simulink model "gm_sfir_fixed_vnl"  (R2021b)
settings: Solver=FixedStepDiscrete  StartTime=0.0  StopTime=2000  RelTol=1e-3
libraries: simulink x2
Description:
  | Symmetric FIR Filter
  | This example shows how to use HDL Coder(TM) to check, generate,
  | and verify HDL for a fixed-point symmetric FIR filter.
settings Model: Creator=The MathWorks, Inc.  LastModifiedBy=Marco Milanesi
settings SolverCC: AlgebraicLoopSolver=TrustRegion
settings DataIOCC: LimitDataPoints=on  SaveFormat=Array  SaveOutput=off  SignalLogging=off  SaveTime=off  ReturnWorkspaceOutputs=off  SignalLoggingName=logsOut
settings OptimizationCC: BlockReduction=off  BooleanDataType=off  ConditionallyExecuteInputs=off  DefaultParameterBehavior=Inlined  InheritOutputTypeSmallerThanSingle=on  InlineInvariantSignals=on  ExpressionDepthLimit=2147483647  InitFltsAndDblsToZero=on  LifeSpan=inf  BufferReusableBoundary=off
settings DebuggingCC: AlgebraicLoopMsg=error  SaveWithParameterizedLinksMsg=none  UnderspecifiedInitializationDetection=Classic  MergeDetectMultiDrivingBlocksExec=none  CheckExecutionContextPreStartOutputMsg=on  SignalResolutionControl=TryResolveAllWithWarning  InheritedTsInSrcMsg=none  MultiTaskDSMMsg=warning  MultiTaskCondExecSysMsg=none  SingleTaskRateTransMsg=error  IntegerOverflowMsg=none  ParameterPrecisionLossMsg=none  FcnCallInpInsideContextMsg=warning  BusObjectLabelMismatch=none  StateNameClashWarn=warning  SFUnexpectedBacktrackingDiag=warning  SFNoUnconditionalDefaultTransitionDiag=warning  SFExecutionAtInitializationDiag=none  SFMachineParentedDataDiag=warning  IntegerSaturationMsg=none  ArithmeticOperatorsInVariantConditions=warning
settings HardwareCC: ProdBitPerPointer=32  ProdBitPerSizeT=32  ProdBitPerPtrDiffT=32  ProdLargestAtomicFloat=None  ProdIntDivRoundTo=Undefined  ProdEndianess=Unspecified  ProdWordSize=32  ProdHWDeviceType=ASIC/FPGA  TargetUnknown=on  ProdEqTarget=off
settings ModelReferenceCC: PropagateSignalLabelsOutOfModel=off
settings SFSimCC: SimUseLocalCustomCode=off  CustomCodeUndefinedFunction=UseInterfaceOnly
settings RTWCC: RTWUseLocalCustomCode=off
settings CodeAppCC: StateflowObjectComments=on
settings GRTTargetCC: TargetFcnLib=ansi_tfl_tmw.mat  TargetLangStandard=C89/C90 (ANSI)  CombineOutputUpdateFcns=off  GRTInterface=on
settings ConfigComp: CovMetricSettings=dw  CovSaveCumulativeToWorkspaceVar=on  CovSaveSingleToWorkspaceVar=on  CovExternalEMLEnable=off

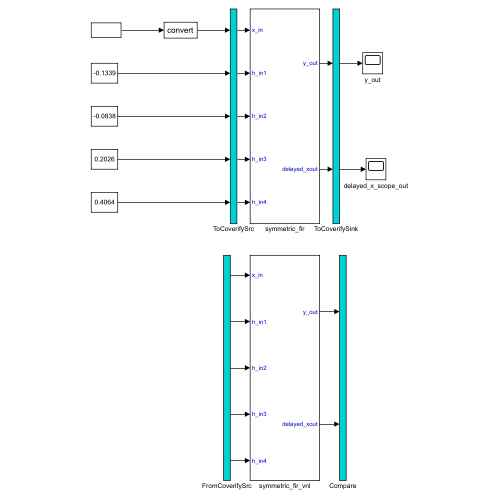
[thumbnail: Simulink's stored preview of the top-level diagram]
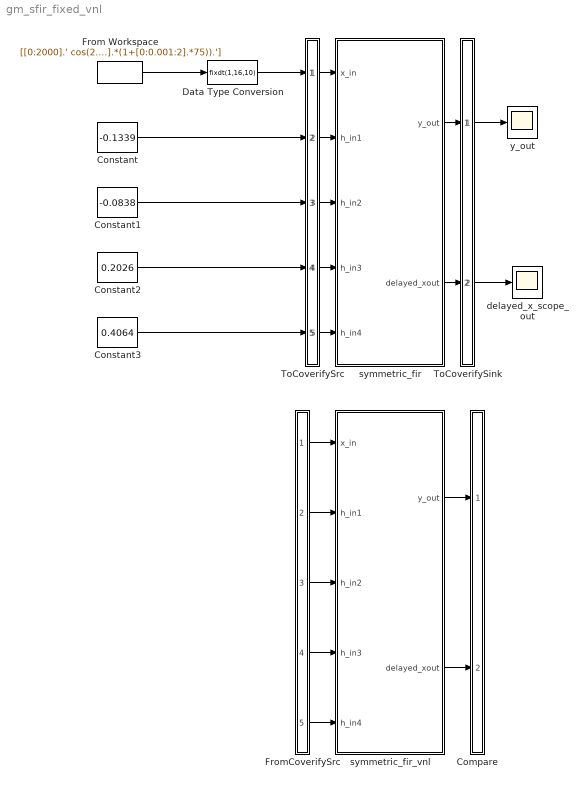
== system gm_sfir_fixed_vnl ==
  Compare : Subsystem
      mask Display: disp('')
  Constant : Constant  Value=-0.1339  OutDataTypeStr=fixdt(1,16,10)  SampleTime=1
  Constant1 : Constant  Value=-0.0838  OutDataTypeStr=fixdt(1,16,10)  SampleTime=1
  Constant2 : Constant  Value=0.2026  OutDataTypeStr=fixdt(1,16,10)  SampleTime=1
  Constant3 : Constant  Value=0.4064  OutDataTypeStr=fixdt(1,16,10)  SampleTime=1
  Data Type Conversion : DataTypeConversion  OutDataTypeStr=fixdt(1,16,10)
  From Workspace : FromWorkspace  VariableName=[[0:2000].' cos(2.*pi.*[0:0.001:2].*(1+[0:0.001:2].*75)).']  SampleTime=1  OutputAfterFinalValue=Setting to zero
  FromCoverifySrc : Subsystem
      mask Display: disp('')
  ToCoverifySink : Subsystem
      mask Display: disp('')
  ToCoverifySrc : Subsystem
      mask Display: disp('')
  delayed_x_scope_out : Scope
  symmetric_fir : Subsystem
  symmetric_fir_vnl : Subsystem
  y_out : Scope
  wires:
  From Workspace/1 -> Data Type Conversion/1
  ToCoverifySrc/1(out1) -> symmetric_fir/1(x_in)
  ToCoverifySrc/2(out2) -> symmetric_fir/2(h_in1)
  ToCoverifySrc/3(out3) -> symmetric_fir/3(h_in2)
  ToCoverifySrc/4(out4) -> symmetric_fir/4(h_in3)
  ToCoverifySrc/5(out5) -> symmetric_fir/5(h_in4)
  symmetric_fir/1(y_out) -> ToCoverifySink/1(in1)
  symmetric_fir/2(delayed_xout) -> ToCoverifySink/2(in2)
  Data Type Conversion/1 -> ToCoverifySrc/1(in1)
  Constant/1 -> ToCoverifySrc/2(in2)
  Constant1/1 -> ToCoverifySrc/3(in3)
  Constant2/1 -> ToCoverifySrc/4(in4)
  Constant3/1 -> ToCoverifySrc/5(in5)
  ToCoverifySink/1(out1) -> y_out/1
  ToCoverifySink/2(out2) -> delayed_x_scope_out/1
  FromCoverifySrc/1(out1) -> symmetric_fir_vnl/1(x_in)
  FromCoverifySrc/2(out2) -> symmetric_fir_vnl/2(h_in1)
  FromCoverifySrc/3(out3) -> symmetric_fir_vnl/3(h_in2)
  FromCoverifySrc/4(out4) -> symmetric_fir_vnl/4(h_in3)
  FromCoverifySrc/5(out5) -> symmetric_fir_vnl/5(h_in4)
  symmetric_fir_vnl/1(y_out) -> Compare/1(in1)
  symmetric_fir_vnl/2(delayed_xout) -> Compare/2(in2)

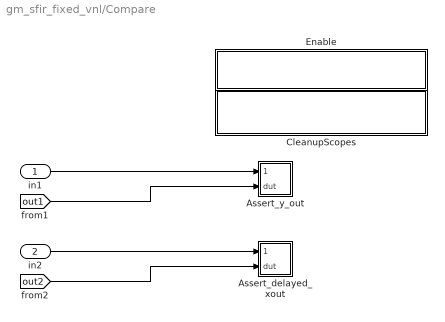
== system gm_sfir_fixed_vnl/Compare ==
  in1 : Inport
  in2 : Inport  Port=2
  Assert_delayed_xout : Subsystem
  Assert_y_out : Subsystem
  CleanupScopes : Subsystem
      settings: OpenFcn=|
      | blkName = gcb; %self block
      | idx = regexp(blkName, '/CleanupScopes$', 'once');
      | blkParent = blkName(1:idx-1);
      | blks=find_system(blkParent, 'LookUnderMasks', 'all','blocktype', 'Scope');
      | for itr = 1:length(blks)
      | 	 hScopeCfg = get_param(blks{itr},'ScopeConfiguration');
      | 	 hScopeCfg.Visible = ~ hScopeCfg.Visible;
      | end
      | drawnow;
      mask Display: fprintf(message('hdlcoder:cosim:vnl_dblclick').getString());
  Enable : Subsystem
      settings: OpenFcn=|
      | blkName = gcb;
      | idx = regexp(blkName, '/Enable$', 'once');
      | blkParent = blkName(1:idx-1);
      | blks=find_system(blkParent, 'LookUnderMasks', 'all','blocktype', 'Assertion');
      | e = get_param(blks{1}, 'Enabled');
      | if strcmp(e, 'on'), f= 'off';, else, f = 'on';, end
      | for ii=1:length(blks), set_param(blks{ii}, 'Enabled', f);, end
      | set_param(gcb, 'MaskDisplay',['fprintf(message(''hdlcoder:cosim:vnl_dblclick_assertions'',','''',upper(e),'''',').getString())']);
      mask Display: fprintf(message('hdlcoder:cosim:vnl_dblclick_assertions','OFF').getString());
  wires:
  in1/1 -> Assert_y_out/1(cosim)
  [out1] -> Assert_y_out/2(dut)
  in2/1 -> Assert_delayed_xout/1(cosim)
  [out2] -> Assert_delayed_xout/2(dut)

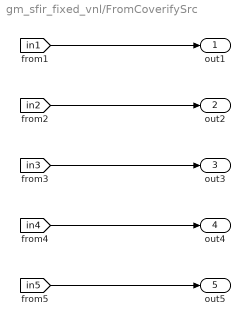
== system gm_sfir_fixed_vnl/FromCoverifySrc ==
  out1 : Outport
  out2 : Outport  Port=2
  out3 : Outport  Port=3
  out4 : Outport  Port=4
  out5 : Outport  Port=5
  wires:
  [in1] -> out1/1
  [in2] -> out2/1
  [in3] -> out3/1
  [in4] -> out4/1
  [in5] -> out5/1

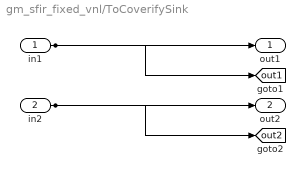
== system gm_sfir_fixed_vnl/ToCoverifySink ==
  in1 : Inport
  in2 : Inport  Port=2
  out1 : Outport
  out2 : Outport  Port=2
  tag scope: out1=global, out2=global
  wires:
  in1/1 -> out1/1, [out1]
  in2/1 -> out2/1, [out2]

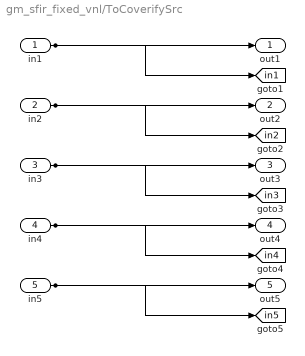
== system gm_sfir_fixed_vnl/ToCoverifySrc ==
  in1 : Inport
  in2 : Inport  Port=2
  in3 : Inport  Port=3
  in4 : Inport  Port=4
  in5 : Inport  Port=5
  out1 : Outport
  out2 : Outport  Port=2
  out3 : Outport  Port=3
  out4 : Outport  Port=4
  out5 : Outport  Port=5
  tag scope: in1=global, in2=global, in3=global, in4=global, in5=global
  wires:
  in1/1 -> out1/1, [in1]
  in2/1 -> out2/1, [in2]
  in3/1 -> out3/1, [in3]
  in4/1 -> out4/1, [in4]
  in5/1 -> out5/1, [in5]

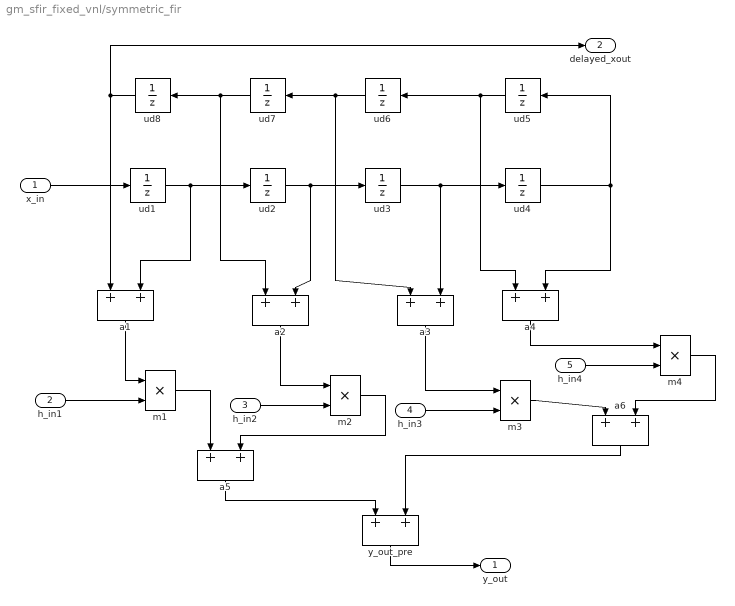
== system gm_sfir_fixed_vnl/symmetric_fir ==
  x_in : Inport
  h_in1 : Inport  Port=2
  h_in2 : Inport  Port=3
  h_in3 : Inport  Port=4
  h_in4 : Inport  Port=5
  a{1..6} (6 alike) : Sum
  m{1..4} (4 alike) : Product  RndMeth=Zero
  ud{1..8} (8 alike) : UnitDelay  SampleTime=-1  HasFrameUpgradeWarning=on
  y_out_pre : Sum
  y_out : Outport  VectorParamsAs1DForOutWhenUnconnected=off
  delayed_xout : Outport  Port=2  VectorParamsAs1DForOutWhenUnconnected=off
  wires:
  a4/1 -> m4/1
  ud7/1 -> a2/1, ud8/1
  ud6/1 -> a3/1, ud7/1
  ud5/1 -> a4/1, ud6/1
  ud2/1 -> a2/2, ud3/1
  ud4/1 -> a4/2, ud5/1
  ud8/1 -> a1/1, delayed_xout/1
  a3/1 -> m3/1
  ud3/1 -> a3/2, ud4/1
  a2/1 -> m2/1
  a1/1 -> m1/1
  m1/1 -> a5/1
  m2/1 -> a5/2
  m3/1 -> a6/1
  m4/1 -> a6/2
  a5/1 -> y_out_pre/1
  a6/1 -> y_out_pre/2
  y_out_pre/1 -> y_out/1
  h_in1/1 -> m1/2
  h_in2/1 -> m2/2
  h_in3/1 -> m3/2
  h_in4/1 -> m4/2
  ud1/1 -> a1/2, ud2/1
  x_in/1 -> ud1/1

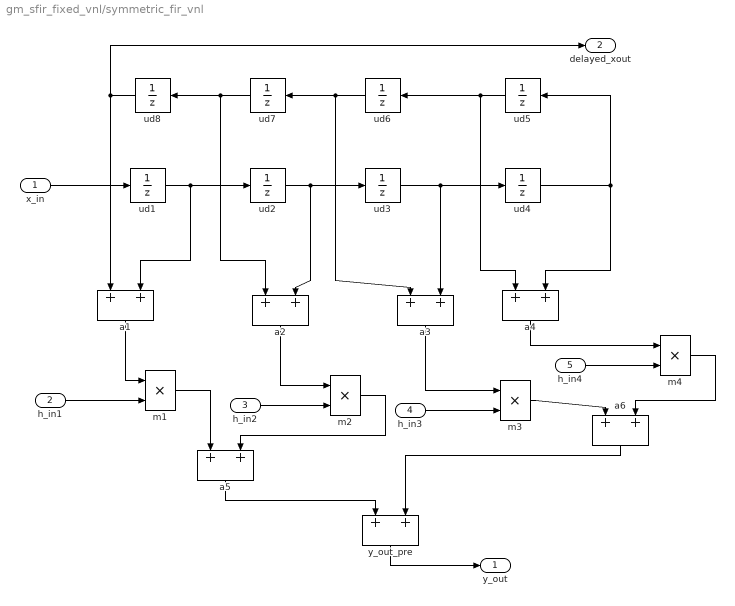
== system gm_sfir_fixed_vnl/symmetric_fir_vnl ==
  x_in : Inport
  h_in1 : Inport  Port=2
  h_in2 : Inport  Port=3
  h_in3 : Inport  Port=4
  h_in4 : Inport  Port=5
  a{1..6} (6 alike) : Sum
  m{1..4} (4 alike) : Product  RndMeth=Zero
  ud{1..8} (8 alike) : UnitDelay  SampleTime=-1  HasFrameUpgradeWarning=on
  y_out_pre : Sum
  y_out : Outport  VectorParamsAs1DForOutWhenUnconnected=off
  delayed_xout : Outport  Port=2  VectorParamsAs1DForOutWhenUnconnected=off
  wires:
  x_in/1 -> ud1/1
  ud1/1 -> ud2/1, a1/2
  h_in4/1 -> m4/2
  h_in3/1 -> m3/2
  h_in2/1 -> m2/2
  h_in1/1 -> m1/2
  y_out_pre/1 -> y_out/1
  a6/1 -> y_out_pre/2
  a5/1 -> y_out_pre/1
  m4/1 -> a6/2
  m3/1 -> a6/1
  m2/1 -> a5/2
  m1/1 -> a5/1
  a1/1 -> m1/1
  a2/1 -> m2/1
  ud3/1 -> ud4/1, a3/2
  a3/1 -> m3/1
  ud8/1 -> delayed_xout/1, a1/1
  ud4/1 -> ud5/1, a4/2
  ud2/1 -> ud3/1, a2/2
  ud5/1 -> ud6/1, a4/1
  ud6/1 -> ud7/1, a3/1
  ud7/1 -> ud8/1, a2/1
  a4/1 -> m4/1

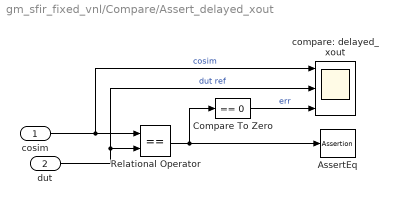
== system gm_sfir_fixed_vnl/Compare/Assert_delayed_xout ==
  cosim : Inport
  dut : Inport  Port=2
  AssertEq : Assertion  StopWhenAssertionFail=off
  Compare To Zero : simulink/Logic and Bit Operations/Compare To Zero  relop===  OutDataTypeStr=boolean
  Relational Operator : RelationalOperator  Operator===  OutDataTypeStr=boolean  RndMeth=Nearest
  compare: delayed_xout : Scope  NumInputPorts=3
  wires:
  Compare To Zero/1 -> compare: delayed_xout/3  "err"
  Relational Operator/1 -> Compare To Zero/1, AssertEq/1
  cosim/1 -> compare: delayed_xout/1, Relational Operator/1  "cosim"
  dut/1 -> compare: delayed_xout/2, Relational Operator/2  "dut ref"

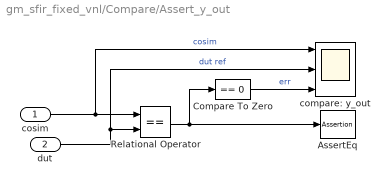
== system gm_sfir_fixed_vnl/Compare/Assert_y_out ==
  cosim : Inport
  dut : Inport  Port=2
  AssertEq : Assertion  StopWhenAssertionFail=off
  Compare To Zero : simulink/Logic and Bit Operations/Compare To Zero  relop===  OutDataTypeStr=boolean
  Relational Operator : RelationalOperator  Operator===  OutDataTypeStr=boolean  RndMeth=Nearest
  compare: y_out : Scope  NumInputPorts=3
  wires:
  Compare To Zero/1 -> compare: y_out/3  "err"
  Relational Operator/1 -> Compare To Zero/1, AssertEq/1
  cosim/1 -> compare: y_out/1, Relational Operator/1  "cosim"
  dut/1 -> compare: y_out/2, Relational Operator/2  "dut ref"

== system gm_sfir_fixed_vnl/Compare/CleanupScopes ==

== system gm_sfir_fixed_vnl/Compare/Enable ==
